simulink model "MRAC_PID_LTI_TEST"  (R2016b)
settings: Solver=VariableStepAuto  StartTime=0.0  StopTime=10.0  RelTol=1e-3
values from neighbouring files (symbols this model uses):
  a0m = omega^2    (= 12.2899097537)    [parameters.m]
  a1m = 2*z*omega    (= 4.90797546012)    [parameters.m]
  a2m = 4    [parameters.m]
  den1 = [1 p q]    [parameters.m]
  den2 = [1 a1m a0m]    [parameters.m]
  gamma_kd = 100    [parameters.m]
  gamma_ki = 20    [parameters.m]
  gamma_kp = 500    [parameters.m]
  num1 = vq2_c(200)    [parameters.m]
  num2 = a0m    (= 12.2899097537)    [parameters.m]
settings Model: Creator=Sarath  LastModifiedBy=Sarath

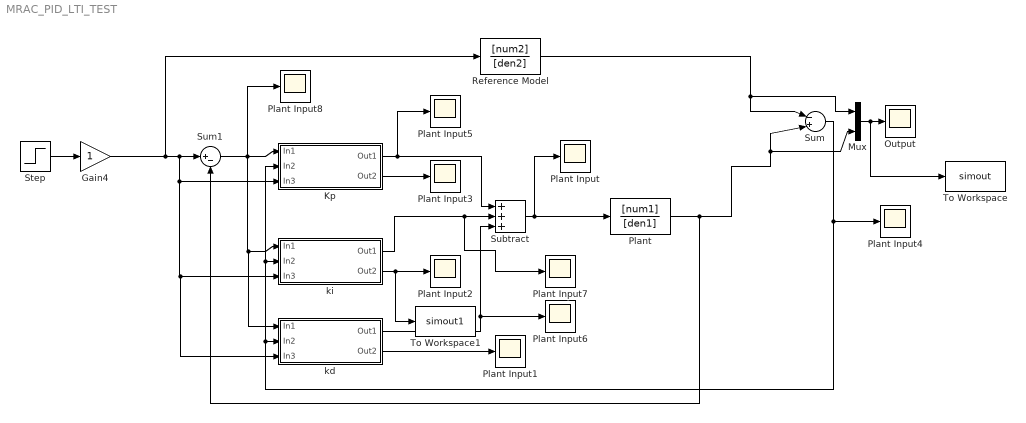
== system MRAC_PID_LTI_TEST ==
  Gain4 : Gain
  "Kp " : Subsystem
  Mux : Mux  Inputs=2
  Output : Scope
  Plant : TransferFcn  Numerator=[num1]  Denominator=[den1]
  Plant Input{,1..8} (9 alike) : Scope
  Reference Model : TransferFcn  Numerator=[num2]  Denominator=[den2]
  Step : Step  Time=0  SampleTime=0
  Subtract : Sum  Inputs=+++
  Sum : Sum  Inputs=|-+|  SaturateOnIntegerOverflow=on
  Sum1 : Sum  Inputs=|+-
  To Workspace : ToWorkspace  VariableName=simout  SaveFormat=Timeseries  SampleTime=-1
  To Workspace1 : ToWorkspace  VariableName=simout1  SaveFormat=Timeseries  SampleTime=-1
  kd : Subsystem
  ki : Subsystem
  wires:
  Reference Model/1 -> Mux/1, Sum/1
  Sum/1 -> Plant Input4/1, "Kp "/2(In2), ki/2(In2), kd/2(In2)
  Mux/1 -> To Workspace/1, Output/1
  Plant/1 -> Sum1/2, Sum/2, Mux/2
  Gain4/1 -> kd/3(In3), ki/3(In3), "Kp "/3(In3), Sum1/1, Reference Model/1
  "Kp "/1(Out1) -> Plant Input5/1, Subtract/1
  kd/1(Out1) -> Plant Input6/1, Subtract/3
  ki/1(Out1) -> Subtract/2, Plant Input7/1
  Subtract/1 -> Plant/1, Plant Input/1
  kd/2(Out2) -> Plant Input1/1
  ki/2(Out2) -> To Workspace1/1, Plant Input2/1
  "Kp "/2(Out2) -> Plant Input3/1
  Step/1 -> Gain4/1
  Sum1/1 -> kd/1(In1), ki/1(In1), Plant Input8/1, "Kp "/1(In1)

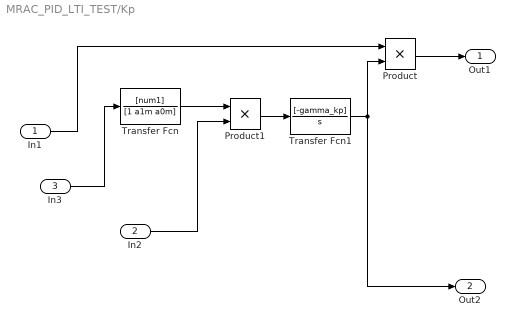
== system MRAC_PID_LTI_TEST/Kp  ==
  In1 : Inport
  In2 : Inport  Port=2
  In3 : Inport  Port=3
  Product : Product
  Product1 : Product
  Transfer Fcn : TransferFcn  Numerator=[num1]  Denominator=[1 a1m a0m]
  Transfer Fcn1 : TransferFcn  Numerator=[-gamma_kp]  Denominator=[1 0]
  Out1 : Outport
  Out2 : Outport  Port=2
  wires:
  In1/1 -> Product/1
  Product/1 -> Out1/1
  Transfer Fcn/1 -> Product1/1
  In2/1 -> Product1/2
  Product1/1 -> Transfer Fcn1/1
  Transfer Fcn1/1 -> Product/2, Out2/1
  In3/1 -> Transfer Fcn/1

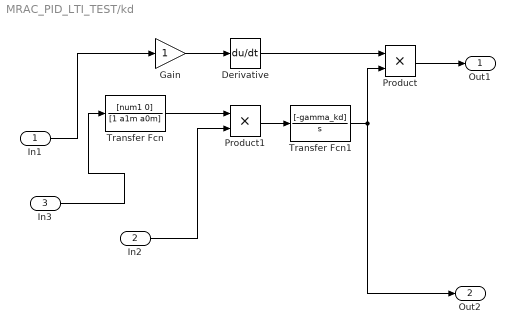
== system MRAC_PID_LTI_TEST/kd ==
  In1 : Inport
  In2 : Inport  Port=2
  In3 : Inport  Port=3
  Derivative : Derivative
  Gain : Gain
  Product : Product
  Product1 : Product
  Transfer Fcn : TransferFcn  Numerator=[num1 0]  Denominator=[1 a1m a0m]
  Transfer Fcn1 : TransferFcn  Numerator=[-gamma_kd]  Denominator=[1 0]
  Out1 : Outport
  Out2 : Outport  Port=2
  wires:
  In1/1 -> Gain/1
  Product/1 -> Out1/1
  Transfer Fcn/1 -> Product1/1
  In2/1 -> Product1/2
  Product1/1 -> Transfer Fcn1/1
  Transfer Fcn1/1 -> Product/2, Out2/1
  Derivative/1 -> Product/1
  Gain/1 -> Derivative/1
  In3/1 -> Transfer Fcn/1

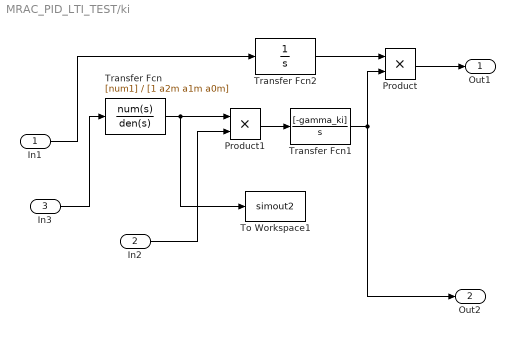
== system MRAC_PID_LTI_TEST/ki ==
  In1 : Inport
  In2 : Inport  Port=2
  In3 : Inport  Port=3
  Product : Product
  Product1 : Product
  To Workspace1 : ToWorkspace  VariableName=simout2  SaveFormat=Timeseries  SampleTime=-1
  Transfer Fcn : TransferFcn  Numerator=[num1]  Denominator=[1 a2m a1m a0m]
  Transfer Fcn1 : TransferFcn  Numerator=[-gamma_ki]  Denominator=[1 0]
  Transfer Fcn2 : TransferFcn  Denominator=[1 0]
  Out1 : Outport
  Out2 : Outport  Port=2
  wires:
  In1/1 -> Transfer Fcn2/1
  Product/1 -> Out1/1
  Transfer Fcn/1 -> Product1/1, To Workspace1/1
  In2/1 -> Product1/2
  Product1/1 -> Transfer Fcn1/1
  Transfer Fcn1/1 -> Product/2, Out2/1
  Transfer Fcn2/1 -> Product/1
  In3/1 -> Transfer Fcn/1
